simulink model "pr5"  (R2016b)
settings: Solver=FixedStepAuto  StartTime=0.0  StopTime=10.0  RelTol=1e-3  EnableMultiTasking=on
libraries: legoev3lib x4, simulink x2
settings Model: ExtModeTrigDuration=2  Creator=Nexel  LastModifiedBy=Nexel
settings SolverCC: PositivePriorityOrder=on
settings OptimizationCC: MaxStackSize=64
settings DebuggingCC: ParameterTunabilityLossMsg=error
settings HardwareCC: ProdBitPerPointer=32  ProdBitPerSizeT=32  ProdBitPerPtrDiffT=32  ProdLargestAtomicInteger=Long  ProdWordSize=32  ProdHWDeviceType=ARM Compatible->ARM 9
settings RTWCC: SystemTargetFile=ert.tlc  HardwareBoard=LEGO MINDSTORMS EV3  TLCOptions="-aInlineSetEventsForThisBaseRateFcn=TLC_FALSE -aSuppressMultiTaskScheduler=TLC_FALSE  -aRateBasedStepFcn=0"  TemplateMakefile=ert_default_tmf  Description=Embedded Coder  GenerateReport=on  Toolchain=Sourcery G++ Lite v2009q3  IncludeHyperlinkInReport=on  LaunchReport=on  GenerateTraceInfo=on  GenerateTraceReport=on  GenerateTraceReportSl=on  GenerateTraceReportSf=on  GenerateTraceReportEml=on
settings CodeAppCC: ForceParamTrailComments=on  IgnoreCustomStorageClasses=off  OperatorAnnotations=on  SimulinkDataObjDesc=on  SFDataObjDesc=on  MATLABFcnDesc=on  InsertBlockDesc=on  MATLABSourceComments=on
settings ERTTargetCC: SupportContinuousTime=on  SupportVariableSizeSignals=on

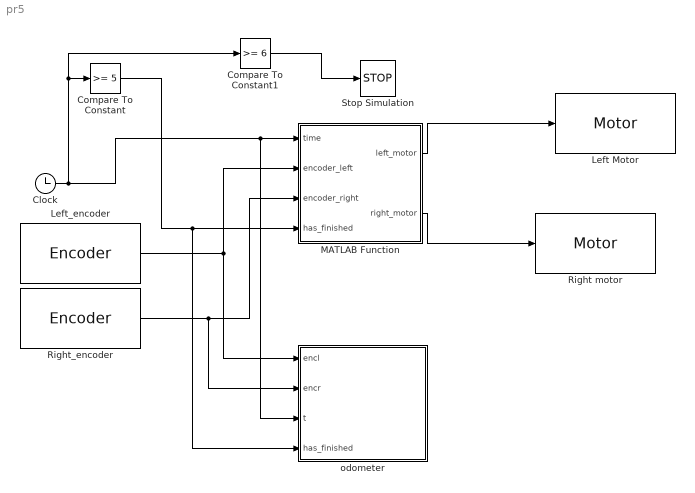
== system pr5 ==
  Clock : Clock
  Compare To Constant : simulink/Logic and Bit Operations/Compare To Constant  relop=>=  const=5  OutDataTypeStr=boolean
  Compare To Constant1 : simulink/Logic and Bit Operations/Compare To Constant  relop=>=  const=6  OutDataTypeStr=boolean
  Left Motor : legoev3lib/Motor  sportNumber=B  sstopAction=Brake
  "Left_encoder " : legoev3lib/Encoder  portNumber=B  opMode=No reset  sampleTime=0.001
  MATLAB Function : MATLAB Function  TreatAsAtomicUnit=on
  "Right motor " : legoev3lib/Motor  sportNumber=C  sstopAction=Brake
  "Right_encoder " : legoev3lib/Encoder  portNumber=C  opMode=No reset  sampleTime=0.001
  Stop Simulation : Stop
  odometer : MATLAB Function  TreatAsAtomicUnit=on
  wires:
  Clock/1 -> odometer/3(t), MATLAB Function/1(time), Compare To Constant1/1, Compare To Constant/1
  MATLAB Function/1(left_motor) -> Left Motor/1
  MATLAB Function/2(right_motor) -> "Right motor "/1
  Compare To Constant/1 -> odometer/4(has_finished), MATLAB Function/4(has_finished)
  "Left_encoder "/1 -> odometer/1(encl), MATLAB Function/2(encoder_left)
  "Right_encoder "/1 -> odometer/2(encr), MATLAB Function/3(encoder_right)
  Compare To Constant1/1 -> Stop Simulation/1

== matlab function pr5/odometer ==
  data: encl input; encr input; t input; has_finished input
function odometer( encl, encr, t, has_finished )

    time  = double(t);
    enc_l = double(encl);
    enc_r = double(encr);

    % define constants
    persistent D R;
    if( isempty(D) )
        D = 0.117;
        R = 0.027;
    end

    % define previous state 
    persistent x0 y0 w0 t0 prev_enc_l prev_enc_r file;
    if( isempty(x0) )
        file = fopen('/home/root/lms2012/prjs/mw/mypose.txt','w');
        x0 = 0;
        y0 = 0;
        w0 = 0;
        t0 = time;
        prev_enc_l = enc_l;
        prev_enc_r = enc_r;
    end
    delta_encl = enc_l - prev_enc_l;
    delta_encr = enc_r - prev_enc_r;
    if(time == t0)
        x1 = 0;
        y1 = 0;
        w1 = 0;
    else
        x1 = ((delta_encl * R + delta_encr * R) / 2) * cosd(w0);
        y1 = ((delta_encl * R + delta_encr * R) / 2) * sind(w0);
        w1 = ((delta_encr * R - delta_encl * R) / D);
    end
    x0 = x0 + x1;
    y0 = y0 + y1;
    w0 = w0 + w1;
    t0 = time;
    prev_enc_l = enc_l;
    prev_enc_r = enc_r;
    fprintf(file,'%f %f %f\n',double(x0), double(y0), double(w0));
    if (has_finished) 
       fclose(file);
    end
end

== matlab function pr5/MATLAB Function ==
  data: time input; left_motor output; right_motor output; encoder_left input; encoder_right input; has_finished input
function [left_motor, right_motor] = fcn(time, encoder_left, encoder_right, has_finished)
    persistent counter;
    persistent isTurning;
    persistent results;
    persistent iteration;
    persistent file;
    if isempty(counter) 
       counter = 0; 
       isTurning = false;
       results = zeros(6,30000);
       iteration = 1;
       file = fopen('/home/root/lms2012/prjs/mw/mylog.txt','w');
    end
    if (isTurning) 
       left_motor = 43;
       right_motor = 0;
    else
        left_motor = 70;
       right_motor = 70;
    end
    results(:,iteration) = [time, encoder_left, encoder_right, 0, 0, 0];
    iteration = iteration + 1;
    if(time - counter > 1) 
       isTurning = ~isTurning;
       counter = time;
    end
    fprintf(file,'%f %f %f\n',double(time), double(encoder_left), double(encoder_right));
    if (has_finished) 
       fclose(file);
    end
end
